simulink model "test_blocks"  (R2019b)
settings: Solver=ode4  StartTime=t_start  StopTime=t_stop  FixedStep=t_step  RelTol=1e-3
undefined symbols (not defined in the file or in its folder): tmp
libraries: dspstat3 x7
settings Model: Creator=Vish  LastModifiedBy=Vish

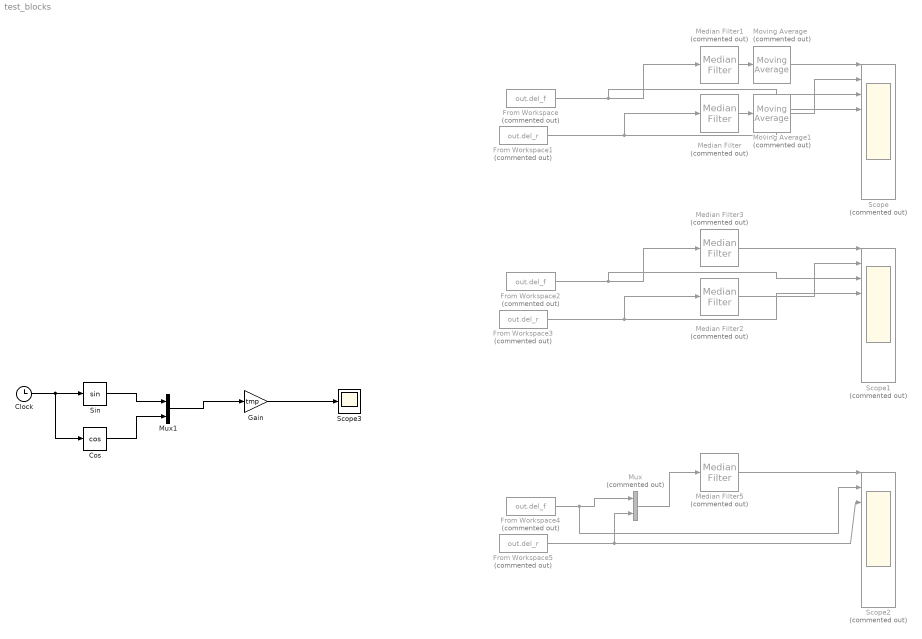
== system test_blocks ==
  Clock : Clock
  Cos : Trigonometry  Operator=cos
  From Workspace : FromWorkspace  Commented=on  VariableName=out.del_f  SampleTime=0
  From Workspace1 : FromWorkspace  Commented=on  VariableName=out.del_r  SampleTime=0
  From Workspace2 : FromWorkspace  Commented=on  VariableName=out.del_f  SampleTime=0
  From Workspace3 : FromWorkspace  Commented=on  VariableName=out.del_r  SampleTime=0
  From Workspace4 : FromWorkspace  Commented=on  VariableName=out.del_f  SampleTime=0
  From Workspace5 : FromWorkspace  Commented=on  VariableName=out.del_r  SampleTime=0
  Gain : Gain  Gain=tmp
  Median Filter : dspstat3/Median Filter  Commented=on  WindowLength=5  SimulateUsing=Interpreted execution
      settings: SourceProductName=DSP System Toolbox  SourceProductBaseCode=DS
  Median Filter1 : dspstat3/Median Filter  Commented=on  WindowLength=5  SimulateUsing=Interpreted execution
      settings: SourceProductName=DSP System Toolbox  SourceProductBaseCode=DS
  Median Filter2 : dspstat3/Median Filter  Commented=on  WindowLength=10  SimulateUsing=Interpreted execution
      settings: SourceProductName=DSP System Toolbox  SourceProductBaseCode=DS
  Median Filter3 : dspstat3/Median Filter  Commented=on  WindowLength=10  SimulateUsing=Interpreted execution
      settings: SourceProductName=DSP System Toolbox  SourceProductBaseCode=DS
  Median Filter5 : dspstat3/Median Filter  Commented=on  WindowLength=10  SimulateUsing=Interpreted execution
      settings: SourceProductName=DSP System Toolbox  SourceProductBaseCode=DS
  Moving Average : dspstat3/Moving Average  Commented=on  Method=Sliding window  ForgettingFactorPort=off  SpecifyWindowLength=on  WindowLength=10  ForgettingFactor=0.9  SimulateUsing=Code generation
  Moving Average1 : dspstat3/Moving Average  Commented=on  Method=Sliding window  ForgettingFactorPort=off  SpecifyWindowLength=on  WindowLength=10  ForgettingFactor=0.9  SimulateUsing=Code generation
  Mux : Mux  Commented=on  Inputs=2
  Mux1 : Mux  Inputs=2
  Scope : Scope  Commented=on  NumInputPorts=10
  Scope1 : Scope  Commented=on  NumInputPorts=10
  Scope2 : Scope  Commented=on  NumInputPorts=10
  Scope3 : Scope
  Sin : Trigonometry
  wires:
  From Workspace/1 -> Scope/3, Median Filter1/1
  From Workspace1/1 -> Scope/4, Median Filter/1
  Median Filter1/1 -> Moving Average/1
  Median Filter/1 -> Moving Average1/1
  Moving Average/1 -> Scope/1
  Moving Average1/1 -> Scope/2
  From Workspace3/1 -> Scope1/4, Median Filter2/1
  Median Filter2/1 -> Scope1/2
  Median Filter3/1 -> Scope1/1
  From Workspace2/1 -> Scope1/3, Median Filter3/1
  Median Filter5/1 -> Scope2/1
  From Workspace4/1 -> Scope2/2, Mux/1
  From Workspace5/1 -> Scope2/3, Mux/2
  Mux/1 -> Median Filter5/1
  Clock/1 -> Cos/1, Sin/1
  Cos/1 -> Mux1/2
  Sin/1 -> Mux1/1
  Mux1/1 -> Gain/1
  Gain/1 -> Scope3/1
